simulink model "Task_33"  (R2022b)
settings: Solver=VariableStepAuto  StartTime=0.0  StopTime=10.0  RelTol=1e-3
settings Model: Creator=Abanob_Sameh  LastModifiedBy=Abanob_Sameh

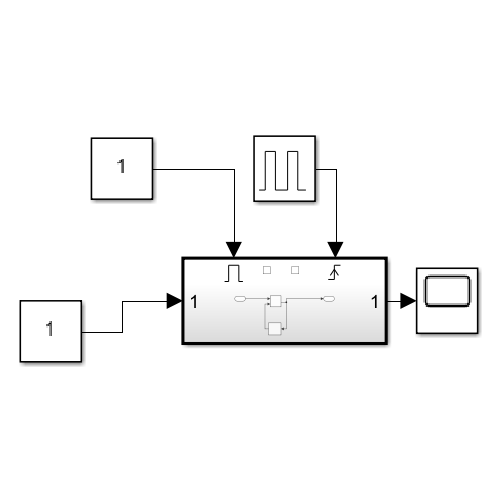
[thumbnail: Simulink's stored preview of the top-level diagram]
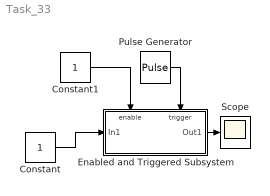
== system Task_33 ==
  Constant : Constant
  Constant1 : Constant
  Enabled and Triggered Subsystem : Subsystem  TreatAsAtomicUnit=on
  Pulse Generator : DiscretePulseGenerator  PulseType=Time based  Period=1  PulseWidth=50
  Scope : Scope
  wires:
  Constant/1 -> Enabled and Triggered Subsystem/1(In1)
  Enabled and Triggered Subsystem/1(Out1) -> Scope/1
  Pulse Generator/1 -> Enabled and Triggered Subsystem/Trigger
  Constant1/1 -> Enabled and Triggered Subsystem/Enable

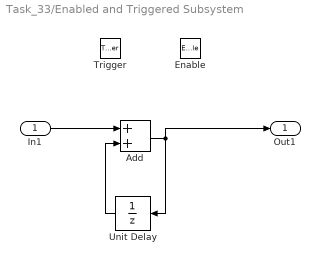
== system Task_33/Enabled and Triggered Subsystem ==
  In1 : Inport
  Enable : EnablePort
  Trigger : TriggerPort  VariantControl=(inherit)
  Add : Sum
  Unit Delay : UnitDelay  SampleTime=-1  HasFrameUpgradeWarning=on
  Out1 : Outport
  wires:
  In1/1 -> Add/1
  Unit Delay/1 -> Add/2
  Add/1 -> Unit Delay/1, Out1/1
